simulink model "FPU_sim1"  (Simulink 7.6)
settings: Solver=FixedStepDiscrete  StartTime=0.0  StopTime=6000  FixedStep=1  RelTol=1e-3
values from neighbouring files (symbols this model uses):
  data_init_sim = zeros(1,100)    [Init_mem.m]    (also in exp_doc.mat = [0 0 0 0 0 0 986822423 3304964096 1146115413 1152155648 1065)
  out_file = [out_file; ['5' buf_oper]]    [Convert_IVE_Program.m]    (also in exp_doc.mat = '78383136191212713131367131313671313136197131361950000000000)
libraries: simulink x50
settings Model: Creator=jordan  LastModifiedBy=jordan
settings OptimizationCC: BlockReduction=off  ConditionallyExecuteInputs=off

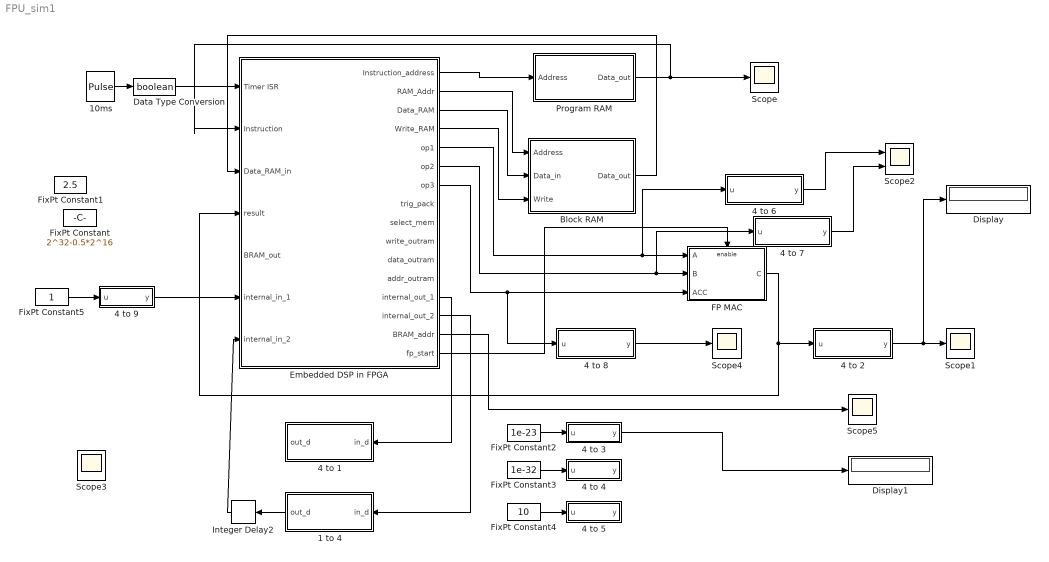
== system FPU_sim1 ==
  1 to 4 : Stateflow chart  TreatAsAtomicUnit=on
  10ms : DiscretePulseGenerator  Period=3000
  4 to 1 : Stateflow chart  TreatAsAtomicUnit=on
  4 to 2 : Stateflow chart  TreatAsAtomicUnit=on
  4 to 3 : Stateflow chart  TreatAsAtomicUnit=on
  4 to 4 : Stateflow chart  TreatAsAtomicUnit=on
  4 to 5 : Stateflow chart  TreatAsAtomicUnit=on
  4 to 6 : Stateflow chart  TreatAsAtomicUnit=on
  4 to 7 : Stateflow chart  TreatAsAtomicUnit=on
  4 to 8 : Stateflow chart  TreatAsAtomicUnit=on
  4 to 9 : Stateflow chart  TreatAsAtomicUnit=on
  Block RAM : Subsystem
  Data Type Conversion : DataTypeConversion  OutDataTypeStr=boolean
  Display : Display
  Display1 : Display
  Embedded DSP in FPGA : Subsystem
  FP MAC : Subsystem
  FixPt Constant : Constant  DisableCoverage=on  Value=2^32-0.5*2^16  OutDataTypeStr=uint32
  FixPt Constant1 : Constant  DisableCoverage=on  Value=2.5  OutDataTypeStr=fixdt(1,32,16)  LockScale=on
  FixPt Constant2 : Constant  DisableCoverage=on  Value=1e-23  OutDataTypeStr=single  LockScale=on
  FixPt Constant3 : Constant  DisableCoverage=on  Value=1e-32  OutDataTypeStr=single  LockScale=on
  FixPt Constant4 : Constant  DisableCoverage=on  Value=10  OutDataTypeStr=single  LockScale=on
  FixPt Constant5 : Constant  DisableCoverage=on  OutDataTypeStr=single  LockScale=on
  Integer Delay2 : simulink/Discrete/Integer Delay  NumDelays=1  vinit=0.0  samptime=-1
  Program RAM : Subsystem
  Scope{,1,3..5} (5 alike) : Scope
      Scope settings: MaxDataPoints=50000
      Scope1 settings: SaveName=ScopeData3  MaxDataPoints=50000
      Scope3 settings: SaveName=ScopeData19  MaxDataPoints=50000
      Scope4 settings: SaveName=ScopeData5  MaxDataPoints=50000
      Scope5 settings: SaveName=ScopeData11  MaxDataPoints=50000
  Scope2 : Scope  NumInputPorts=2
      settings: YMin=-5~-5  YMax=5~5  SaveName=ScopeData4  MaxDataPoints=50000
  wires:
  10ms/1 -> Data Type Conversion/1
  Program RAM/1(Data_out) -> Scope/1, Embedded DSP in FPGA/2(Instruction)
  1 to 4/1(out_d) -> Integer Delay2/1
  Data Type Conversion/1 -> Embedded DSP in FPGA/1(Timer ISR)
  Block RAM/1(Data_out) -> Embedded DSP in FPGA/3(Data_RAM_in)
  Embedded DSP in FPGA/13(internal_out_1) -> 4 to 1/1(in_d)
  Embedded DSP in FPGA/14(internal_out_2) -> 1 to 4/1(in_d)
  Integer Delay2/1 -> Embedded DSP in FPGA/7(internal_in_2)
  Embedded DSP in FPGA/1(Instruction_address) -> Program RAM/1(Address)
  Embedded DSP in FPGA/2(RAM_Addr) -> Block RAM/1(Address)
  Embedded DSP in FPGA/3(Data_RAM) -> Block RAM/2(Data_in)
  Embedded DSP in FPGA/4(Write_RAM) -> Block RAM/3(Write)
  Embedded DSP in FPGA/5(op1) -> 4 to 6/1(u), FP MAC/1(A)
  Embedded DSP in FPGA/6(op2) -> FP MAC/2(B), 4 to 7/1(u)
  Embedded DSP in FPGA/7(op3) -> FP MAC/3(ACC), 4 to 8/1(u)
  FP MAC/1(C) -> Embedded DSP in FPGA/4(result), 4 to 2/1(u)
  4 to 2/1(y) -> Scope1/1, Display/1
  FixPt Constant2/1 -> 4 to 3/1(u)
  4 to 3/1(y) -> Display1/1
  FixPt Constant3/1 -> 4 to 4/1(u)
  FixPt Constant4/1 -> 4 to 5/1(u)
  4 to 6/1(y) -> Scope2/1
  4 to 7/1(y) -> Scope2/2
  4 to 8/1(y) -> Scope4/1
  4 to 9/1(y) -> Embedded DSP in FPGA/6(internal_in_1)
  FixPt Constant5/1 -> 4 to 9/1(u)
  Embedded DSP in FPGA/16(fp_start) -> FP MAC/Enable
  Embedded DSP in FPGA/15(BRAM_addr) -> Scope5/1

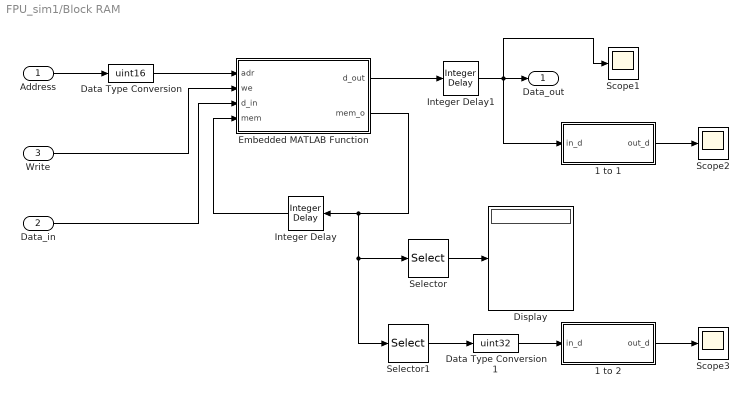
== system FPU_sim1/Block RAM ==
  Address : Inport  OutDataTypeStr=fixdt(0,12,0)
  Data_in : Inport  Port=2  OutDataTypeStr=uint32
  Write : Inport  Port=3  OutDataTypeStr=boolean
  1 to 1 : Stateflow chart  TreatAsAtomicUnit=on
  1 to 2 : Stateflow chart  TreatAsAtomicUnit=on
  Data Type Conversion : DataTypeConversion  OutDataTypeStr=uint16
  Data Type Conversion1 : DataTypeConversion  OutDataTypeStr=uint32
  Display : Display
  Embedded MATLAB Function : Stateflow chart  TreatAsAtomicUnit=on
  Integer Delay : simulink/Discrete/Integer Delay  NumDelays=1  vinit=data_init_sim  samptime=-1
  Integer Delay1 : simulink/Discrete/Integer Delay  NumDelays=1  vinit=0.0  samptime=-1
  Scope1 : Scope
      settings: SaveName=ScopeData23  MaxDataPoints=50000
  Scope2 : Scope
      settings: SaveName=ScopeData14  MaxDataPoints=50000
  Scope3 : Scope
      settings: SaveName=ScopeData31  MaxDataPoints=50000
  Selector : Selector  InputPortWidth=2048  IndexOptions=Index vector (dialog)  Indices=1:5  OutputSizes=1
  Selector1 : Selector  InputPortWidth=2048  IndexOptions=Index vector (dialog)  Indices=37  OutputSizes=1
  Data_out : Outport  OutDataTypeStr=uint32
  wires:
  Address/1 -> Data Type Conversion/1
  Write/1 -> Embedded MATLAB Function/2(we)
  Data_in/1 -> Embedded MATLAB Function/3(d_in)
  Embedded MATLAB Function/1(d_out) -> Integer Delay1/1
  Integer Delay/1 -> Embedded MATLAB Function/4(mem)
  Embedded MATLAB Function/2(mem_o) -> Integer Delay/1, Selector/1, Selector1/1
  Data Type Conversion/1 -> Embedded MATLAB Function/1(adr)
  Integer Delay1/1 -> Data_out/1, Scope1/1, 1 to 1/1(in_d)
  Selector/1 -> Display/1
  1 to 1/1(out_d) -> Scope2/1
  1 to 2/1(out_d) -> Scope3/1
  Selector1/1 -> Data Type Conversion1/1
  Data Type Conversion1/1 -> 1 to 2/1(in_d)

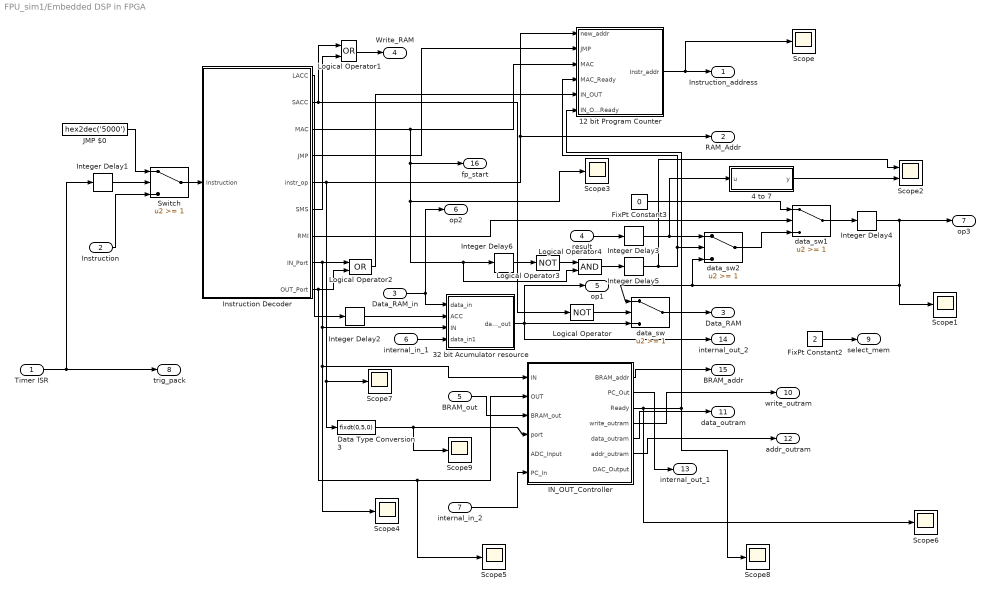
== system FPU_sim1/Embedded DSP in FPGA ==
  Timer ISR : Inport  OutDataTypeStr=boolean
  Instruction : Inport  Port=2  OutDataTypeStr=uint16
  Data_RAM_in : Inport  Port=3  OutDataTypeStr=uint32
  result : Inport  Port=4  OutDataTypeStr=uint32
  BRAM_out : Inport  Port=5  OutDataTypeStr=uint8
  internal_in_1 : Inport  Port=6  OutDataTypeStr=uint32
  internal_in_2 : Inport  Port=7  OutDataTypeStr=uint8  PortDimensions=4
  12 bit Program Counter : Subsystem
  32 bit Acumulator resource : Subsystem
  4 to 7 : Stateflow chart  TreatAsAtomicUnit=on
  Data Type Conversion3 : DataTypeConversion  OutDataTypeStr=fixdt(0,5,0)
  FixPt Constant2 : Constant  DisableCoverage=on  Value=2  OutDataTypeStr=fixdt(0,4,0)
  FixPt Constant3 : Constant  DisableCoverage=on  Value=0  OutDataTypeStr=uint32
  IN_OUT_Controller : Subsystem
  Instruction Decoder : Subsystem
  Integer Delay{1..4,6} (5 alike) : simulink/Discrete/Integer Delay  NumDelays=1  vinit=0.0  samptime=-1
  Integer Delay5 : simulink/Discrete/Integer Delay  NumDelays=3  vinit=0.0  samptime=-1
  JMP $0 : Constant  DisableCoverage=on  Value=hex2dec('5000')  OutDataTypeStr=Inherit: Inherit via back propagation
  Logical Operator : Logic  Operator=NOT  AllPortsSameDT=off  OutDataTypeStr=boolean
  Logical Operator1 : Logic  Operator=OR  AllPortsSameDT=off  OutDataTypeStr=boolean
  Logical Operator2 : Logic  Operator=OR  AllPortsSameDT=off  OutDataTypeStr=boolean
  Logical Operator3 : Logic  Operator=NOT  AllPortsSameDT=off  OutDataTypeStr=boolean
  Logical Operator4 : Logic  AllPortsSameDT=off  OutDataTypeStr=boolean
  Scope{,1,3..9} (9 alike) : Scope
      Scope settings: YMin=0  YMax=650  SaveName=ScopeData2  MaxDataPoints=50000
      Scope1 settings: SaveName=ScopeData6  MaxDataPoints=50000
      Scope3 settings: SaveName=ScopeData8  MaxDataPoints=50000
      Scope4 settings: SaveName=ScopeData10  MaxDataPoints=50000
      Scope5 settings: SaveName=ScopeData21  MaxDataPoints=50000
      Scope6 settings: SaveName=ScopeData13  MaxDataPoints=50000
      Scope7 settings: SaveName=ScopeData15  MaxDataPoints=50000
      Scope8 settings: SaveName=ScopeData16  MaxDataPoints=50000
      Scope9 settings: SaveName=ScopeData12  MaxDataPoints=50000
  Scope2 : Scope  NumInputPorts=2
      settings: YMin=-5~-5  YMax=5~5  SaveName=ScopeData7  MaxDataPoints=50000
  Switch : Switch  Threshold=1
  data_sw : Switch  Threshold=1
  data_sw1 : Switch  Threshold=1
  data_sw2 : Switch  Threshold=1
  Instruction_address : Outport  OutDataTypeStr=fixdt(0,12,0)
  RAM_Addr : Outport  Port=2  OutDataTypeStr=fixdt(0,12,0)
  Data_RAM : Outport  Port=3  OutDataTypeStr=uint32
  Write_RAM : Outport  Port=4  OutDataTypeStr=boolean
  op1 : Outport  Port=5  OutDataTypeStr=uint32
  op2 : Outport  Port=6  OutDataTypeStr=uint32
  op3 : Outport  Port=7  OutDataTypeStr=uint32
  trig_pack : Outport  Port=8
  select_mem : Outport  Port=9
  write_outram : Outport  Port=10
  data_outram : Outport  Port=11
  addr_outram : Outport  Port=12
  internal_out_1 : Outport  Port=13
  internal_out_2 : Outport  Port=14  OutDataTypeStr=uint32
  BRAM_addr : Outport  Port=15
  fp_start : Outport  Port=16  OutDataTypeStr=boolean
  wires:
  32 bit Acumulator resource/1(data_out) -> data_sw/3, op1/1, internal_out_2/1
  Data_RAM_in/1 -> 32 bit Acumulator resource/1(data_in), op2/1
  Instruction Decoder/5(instr_op) -> 12 bit Program Counter/1(new_addr), RAM_Addr/1, Data Type Conversion3/1, Scope7/1
  Instruction Decoder/1(LACC) -> Integer Delay2/1
  Integer Delay2/1 -> 32 bit Acumulator resource/2(ACC)
  Instruction Decoder/2(SACC) -> Logical Operator/1, Logical Operator1/1
  Logical Operator/1 -> data_sw/2
  Instruction Decoder/4(JMP) -> 12 bit Program Counter/2(JMP)
  Instruction Decoder/3(MAC) -> 12 bit Program Counter/3(MAC), fp_start/1, Logical Operator4/2, Integer Delay6/1, Scope3/1
  Instruction Decoder/7(RMI) -> data_sw1/2
  Instruction Decoder/6(SMS) -> Logical Operator1/2
  Instruction Decoder/8(IN_Port) -> 32 bit Acumulator resource/3(IN), Scope4/1, IN_OUT_Controller/1(IN), Logical Operator2/1
  Data Type Conversion3/1 -> Scope9/1, IN_OUT_Controller/4(port)
  Switch/1 -> Instruction Decoder/1(Instruction)
  JMP $0/1 -> Switch/1
  12 bit Program Counter/1(Instr_addr) -> Instruction_address/1, Scope/1
  Instruction/1 -> Switch/3
  data_sw/1 -> Data_RAM/1
  Logical Operator1/1 -> Write_RAM/1
  result/1 -> Integer Delay3/1
  Instruction Decoder/9(OUT_Port) -> Logical Operator2/2, Scope5/1, IN_OUT_Controller/2(OUT)
  IN_OUT_Controller/4(write_outram) -> write_outram/1
  IN_OUT_Controller/5(data_outram) -> data_outram/1
  IN_OUT_Controller/3(Ready) -> 12 bit Program Counter/6(IN_OUT_Ready), Scope8/1, Scope6/1
  Logical Operator2/1 -> 12 bit Program Counter/5(IN_OUT)
  internal_in_1/1 -> 32 bit Acumulator resource/4(data_in1)
  internal_in_2/1 -> IN_OUT_Controller/6(PC_In)
  Integer Delay1/1 -> Switch/2
  IN_OUT_Controller/2(PC_Out) -> internal_out_1/1
  IN_OUT_Controller/1(BRAM_addr) -> BRAM_addr/1
  FixPt Constant2/1 -> select_mem/1
  Timer ISR/1 -> trig_pack/1, Integer Delay1/1
  Integer Delay4/1 -> data_sw2/3, data_sw/1, Scope1/1, op3/1
  data_sw1/1 -> Integer Delay4/1
  FixPt Constant3/1 -> data_sw1/1
  data_sw2/1 -> data_sw1/3
  Integer Delay3/1 -> data_sw2/1, 4 to 7/1(u)
  4 to 7/1(y) -> Scope2/2
  Integer Delay5/1 -> 12 bit Program Counter/4(MAC_Ready), data_sw2/2, Scope2/1
  Integer Delay6/1 -> Logical Operator3/1
  Logical Operator3/1 -> Logical Operator4/1
  Logical Operator4/1 -> Integer Delay5/1
  IN_OUT_Controller/6(addr_outram) -> addr_outram/1
  BRAM_out/1 -> IN_OUT_Controller/3(BRAM_out)

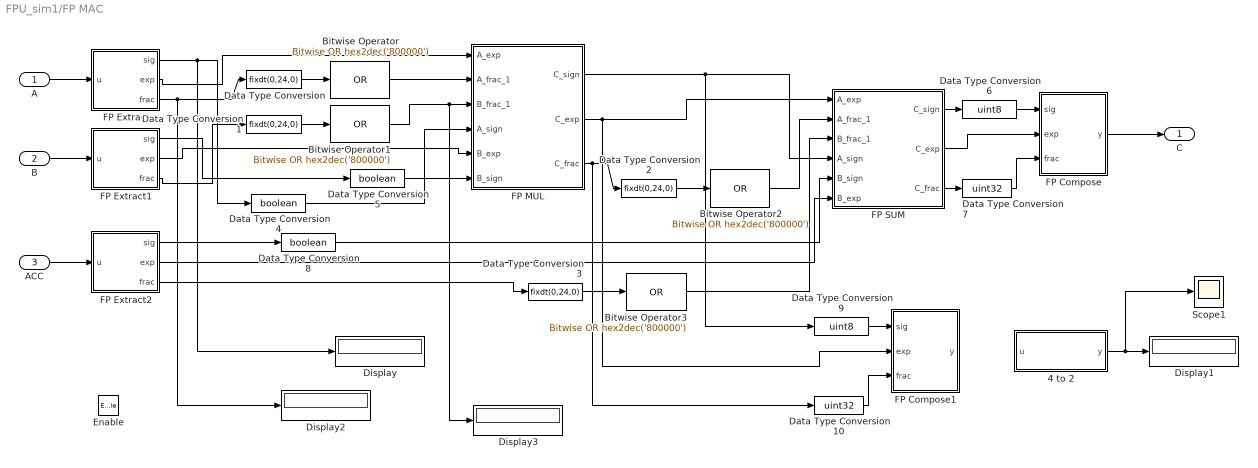
== system FPU_sim1/FP MAC ==
  A : Inport
  B : Inport  Port=2
  ACC : Inport  Port=3
  Enable : EnablePort
  4 to 2 : Stateflow chart  TreatAsAtomicUnit=on
  Bitwise Operator{,1..3} (4 alike) : simulink/Logic and Bit Operations/Bitwise Operator  logicop=OR  UseBitMask=on  BitMask=hex2dec('800000')  BitMaskRealWorld=Stored Integer
  Data Type Conversion{,1..3} (4 alike) : DataTypeConversion  OutDataTypeStr=fixdt(0,24,0)  RndMeth=Nearest
  Data Type Conversion10 : DataTypeConversion  OutDataTypeStr=uint32  RndMeth=Nearest
  Data Type Conversion4 : DataTypeConversion  OutDataTypeStr=boolean  RndMeth=Nearest
  Data Type Conversion5 : DataTypeConversion  OutDataTypeStr=boolean  RndMeth=Nearest
  Data Type Conversion6 : DataTypeConversion  OutDataTypeStr=uint8  RndMeth=Nearest
  Data Type Conversion7 : DataTypeConversion  OutDataTypeStr=uint32  RndMeth=Nearest
  Data Type Conversion8 : DataTypeConversion  OutDataTypeStr=boolean  RndMeth=Nearest
  Data Type Conversion9 : DataTypeConversion  OutDataTypeStr=uint8  RndMeth=Nearest
  Display{,1..3} (4 alike) : Display
      Display3 settings: Format=hex (Stored Integer)
  FP Compose : Stateflow chart  TreatAsAtomicUnit=on
  FP Compose1 : Stateflow chart  TreatAsAtomicUnit=on
  FP Extract : Stateflow chart  TreatAsAtomicUnit=on
  FP Extract1 : Stateflow chart  TreatAsAtomicUnit=on
  FP Extract2 : Stateflow chart  TreatAsAtomicUnit=on
  FP MUL : Subsystem
  FP SUM : Subsystem
  Scope1 : Scope
      settings: SaveName=ScopeData9  MaxDataPoints=50000
  C : Outport  InitialOutput=0
  wires:
  A/1 -> FP Extract/1(u)
  B/1 -> FP Extract1/1(u)
  ACC/1 -> FP Extract2/1(u)
  FP Extract/1(sig) -> Data Type Conversion4/1, Display/1
  FP Extract1/1(sig) -> Data Type Conversion5/1
  FP Extract/2(exp) -> FP MUL/1(A_exp)
  FP Extract1/2(exp) -> FP MUL/5(B_exp)
  FP Extract/3(frac) -> Data Type Conversion/1, Display2/1
  FP Extract1/3(frac) -> Data Type Conversion1/1
  Data Type Conversion/1 -> Bitwise Operator/1
  Bitwise Operator/1 -> FP MUL/2(A_frac_1)
  Data Type Conversion1/1 -> Bitwise Operator1/1
  Bitwise Operator1/1 -> FP MUL/3(B_frac_1), Display3/1
  FP MUL/1(C_sign) -> FP SUM/4(A_sign), Data Type Conversion9/1
  FP MUL/2(C_exp) -> FP SUM/1(A_exp), FP Compose1/2(exp)
  FP MUL/3(C_frac) -> Data Type Conversion2/1, Data Type Conversion10/1
  Data Type Conversion2/1 -> Bitwise Operator2/1
  Bitwise Operator2/1 -> FP SUM/2(A_frac_1)
  FP Extract2/1(sig) -> Data Type Conversion8/1
  FP Extract2/2(exp) -> FP SUM/6(B_exp)
  FP Extract2/3(frac) -> Data Type Conversion3/1
  Data Type Conversion3/1 -> Bitwise Operator3/1
  Bitwise Operator3/1 -> FP SUM/3(B_frac_1)
  Data Type Conversion4/1 -> FP MUL/4(A_sign)
  Data Type Conversion5/1 -> FP MUL/6(B_sign)
  FP SUM/1(C_sign) -> Data Type Conversion6/1
  FP SUM/2(C_exp) -> FP Compose/2(exp)
  FP SUM/3(C_frac) -> Data Type Conversion7/1
  FP Compose/1(y) -> C/1
  Data Type Conversion6/1 -> FP Compose/1(sig)
  Data Type Conversion7/1 -> FP Compose/3(frac)
  Data Type Conversion8/1 -> FP SUM/5(B_sign)
  Data Type Conversion9/1 -> FP Compose1/1(sig)
  Data Type Conversion10/1 -> FP Compose1/3(frac)
  4 to 2/1(y) -> Display1/1, Scope1/1

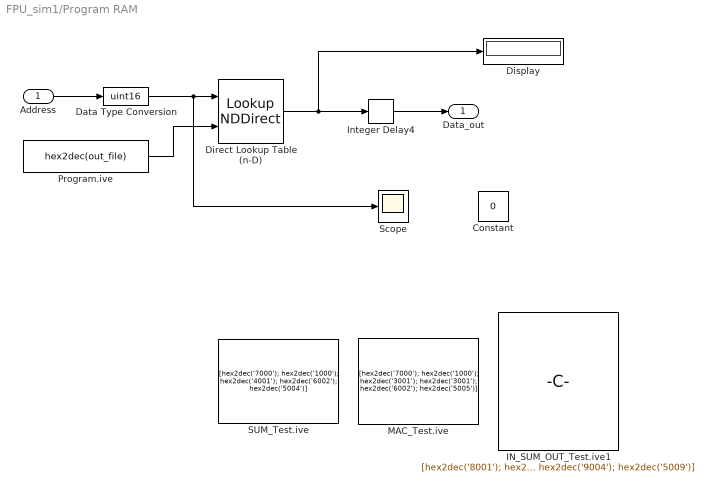
== system FPU_sim1/Program RAM ==
  Address : Inport
  Constant : Constant  Value=0
  Data Type Conversion : DataTypeConversion  OutDataTypeStr=uint16
  Direct Lookup Table (n-D) : LookupNDDirect  NumberOfTableDimensions=1  TableIsInput=on  Table=[hex2dec('1000') hex2dec('4001') hex2dec('2002') hex2dec('5003')]  SampleTime=1  TableDataTypeStr=uint16
  Display : Display
      settings: Format=hex (Stored Integer)
  IN_SUM_OUT_Test.ive1 : Constant  Value=[hex2dec('8001'); hex2dec('2000'); hex2dec('8002'); hex2dec('2001'); hex2dec('1000'); hex2dec('4001'); hex2dec('6002'); hex2dec('1002'); hex2dec('9004'); hex2dec('5009')]  VectorParams1D=off  OutDataTypeStr=uint16
  Integer Delay4 : simulink/Discrete/Integer Delay  NumDelays=1  vinit=0.0  samptime=-1
  MAC_Test.ive : Constant  Value=[hex2dec('7000'); hex2dec('1000'); hex2dec('3001'); hex2dec('3001'); hex2dec('6002'); hex2dec('5005')]  VectorParams1D=off  OutDataTypeStr=uint16
  Program.ive : Constant  Value=hex2dec(out_file)  VectorParams1D=off  OutDataTypeStr=uint16
  SUM_Test.ive : Constant  Value=[hex2dec('7000'); hex2dec('1000'); hex2dec('4001'); hex2dec('6002'); hex2dec('5004')]  VectorParams1D=off  OutDataTypeStr=uint16
  Scope : Scope
      settings: MaxDataPoints=50000
  Data_out : Outport
  wires:
  Address/1 -> Data Type Conversion/1
  Direct Lookup Table (n-D)/1 -> Display/1, Integer Delay4/1
  Program.ive/1 -> Direct Lookup Table (n-D)/2
  Integer Delay4/1 -> Data_out/1
  Data Type Conversion/1 -> Direct Lookup Table (n-D)/1, Scope/1

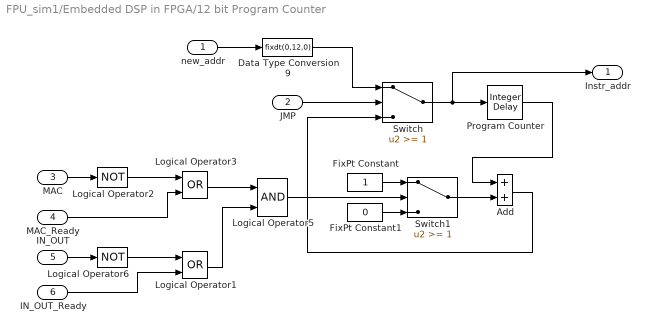
== system FPU_sim1/Embedded DSP in FPGA/12 bit Program Counter ==
  new_addr : Inport
  JMP : Inport  Port=2
  MAC : Inport  Port=3  OutDataTypeStr=boolean
  MAC_Ready : Inport  Port=4  OutDataTypeStr=boolean
  IN_OUT : Inport  Port=5  OutDataTypeStr=boolean
  IN_OUT_Ready : Inport  Port=6  OutDataTypeStr=boolean
  Add : Sum  AccumDataTypeStr=fixdt(0,12,0)  OutDataTypeStr=fixdt(0,12,0)
  Data Type Conversion9 : DataTypeConversion  OutDataTypeStr=fixdt(0,12,0)
  FixPt Constant : Constant  DisableCoverage=on  OutDataTypeStr=fixdt(0,12,0)
  FixPt Constant1 : Constant  DisableCoverage=on  Value=0  OutDataTypeStr=fixdt(0,12,0)
  Logical Operator1 : Logic  Operator=OR  AllPortsSameDT=off  OutDataTypeStr=boolean
  Logical Operator2 : Logic  Operator=NOT  AllPortsSameDT=off  OutDataTypeStr=boolean
  Logical Operator3 : Logic  Operator=OR  AllPortsSameDT=off  OutDataTypeStr=boolean
  Logical Operator5 : Logic  AllPortsSameDT=off  OutDataTypeStr=boolean
  Logical Operator6 : Logic  Operator=NOT  AllPortsSameDT=off  OutDataTypeStr=boolean
  Program Counter : simulink/Discrete/Integer Delay  NumDelays=1  vinit=0.0  samptime=-1
  Switch : Switch  Threshold=1
  Switch1 : Switch  Threshold=1
  Instr_addr : Outport  InitialOutput=0
  wires:
  JMP/1 -> Switch/2
  new_addr/1 -> Data Type Conversion9/1
  Program Counter/1 -> Add/1
  Switch/1 -> Program Counter/1, Instr_addr/1
  FixPt Constant/1 -> Switch1/1
  Add/1 -> Switch/3
  Data Type Conversion9/1 -> Switch/1
  Switch1/1 -> Add/2
  FixPt Constant1/1 -> Switch1/3
  Logical Operator3/1 -> Logical Operator5/1
  Logical Operator2/1 -> Logical Operator3/1
  MAC/1 -> Logical Operator2/1
  Logical Operator1/1 -> Logical Operator5/2
  Logical Operator6/1 -> Logical Operator1/1
  IN_OUT/1 -> Logical Operator6/1
  IN_OUT_Ready/1 -> Logical Operator1/2
  Logical Operator5/1 -> Switch1/2
  MAC_Ready/1 -> Logical Operator3/2

== system FPU_sim1/Embedded DSP in FPGA/32 bit Acumulator resource ==
  data_in : Inport
  ACC : Inport  Port=2
  IN : Inport  Port=3
  data_in1 : Inport  Port=4
  Integer Delay2 : simulink/Discrete/Integer Delay  NumDelays=1  vinit=0.0  samptime=-1
  Switch : Switch  Threshold=1
  Switch1 : Switch  Threshold=1
  data_out : Outport  OutDataTypeStr=uint32
  wires:
  Switch/1 -> Switch1/3
  Integer Delay2/1 -> Switch/3
  data_in/1 -> Switch/1
  ACC/1 -> Switch/2
  Switch1/1 -> Integer Delay2/1, data_out/1
  IN/1 -> Switch1/2
  data_in1/1 -> Switch1/1

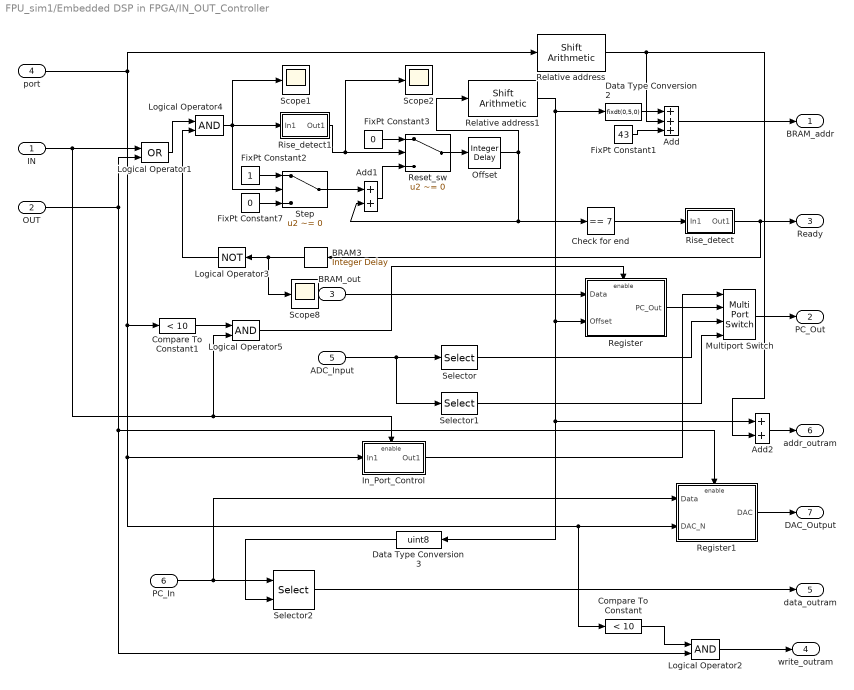
== system FPU_sim1/Embedded DSP in FPGA/IN_OUT_Controller ==
  IN : Inport  OutDataTypeStr=boolean
  OUT : Inport  Port=2  OutDataTypeStr=boolean
  BRAM_out : Inport  Port=3  OutDataTypeStr=uint8
  port : Inport  Port=4  OutDataTypeStr=fixdt(0,5,0)
  ADC_Input : Inport  Port=5  OutDataTypeStr=uint8  PortDimensions=8
  PC_In : Inport  Port=6  OutDataTypeStr=uint8  PortDimensions=4
  Add : Sum  Inputs=+++  AccumDataTypeStr=fixdt(0,11,0)  OutDataTypeStr=fixdt(0,11,0)  SaturateOnIntegerOverflow=on
  Add1 : Sum  AccumDataTypeStr=fixdt(0,3,0)  OutDataTypeStr=fixdt(0,3,0)  SaturateOnIntegerOverflow=on
  Add2 : Sum  AccumDataTypeStr=fixdt(0,14,0)  OutDataTypeStr=fixdt(0,14,0)
  BRAM3 : simulink/Discrete/Integer Delay  NumDelays=1  vinit=0.0  samptime=-1
  Check for end : simulink/Logic and Bit Operations/Compare To Constant  SystemSampleTime=-1  relop===  const=7  LogicOutDataTypeMode=boolean
  Compare To Constant : simulink/Logic and Bit Operations/Compare To Constant  SystemSampleTime=-1  relop=<  const=10  LogicOutDataTypeMode=boolean
  Compare To Constant1 : simulink/Logic and Bit Operations/Compare To Constant  SystemSampleTime=-1  relop=<  const=10  LogicOutDataTypeMode=boolean
  Data Type Conversion2 : DataTypeConversion  OutDataTypeStr=fixdt(0,5,0)
  Data Type Conversion3 : DataTypeConversion  OutDataTypeStr=uint8
  FixPt Constant1 : Constant  DisableCoverage=on  Value=43  OutDataTypeStr=fixdt(0,11,0)
  FixPt Constant2 : Constant  DisableCoverage=on  OutDataTypeStr=fixdt(0,3,0)
  FixPt Constant3 : Constant  DisableCoverage=on  Value=0  OutDataTypeStr=fixdt(0,3,0)
  FixPt Constant7 : Constant  DisableCoverage=on  Value=0  OutDataTypeStr=fixdt(0,3,0)
  In_Port_Control : Subsystem
  Logical Operator1 : Logic  Operator=OR  AllPortsSameDT=off  OutDataTypeStr=boolean
  Logical Operator2 : Logic  AllPortsSameDT=off  OutDataTypeStr=boolean
  Logical Operator3 : Logic  Operator=NOT  AllPortsSameDT=off  OutDataTypeStr=boolean
  Logical Operator4 : Logic  AllPortsSameDT=off  OutDataTypeStr=boolean
  Logical Operator5 : Logic  AllPortsSameDT=off  OutDataTypeStr=boolean
  Multiport Switch : MultiPortSwitch  DataPortOrder=Zero-based contiguous  zeroidx=on
  Offset : simulink/Discrete/Integer Delay  NumDelays=1  vinit=0.0  samptime=0
  Register : Subsystem
  Register1 : Subsystem
  Relative address : simulink/Logic and Bit Operations/Shift Arithmetic  SystemSampleTime=-1  nBitShiftRight=-2  nBinPtShiftRight=0
  Relative address1 : simulink/Logic and Bit Operations/Shift Arithmetic  SystemSampleTime=-1  nBitShiftRight=1  nBinPtShiftRight=0
  Reset_sw : Switch  Criteria=u2 ~= 0
  Rise_detect : Subsystem
  Rise_detect1 : Subsystem
  Scope1 : Scope
      settings: SaveName=ScopeData18  MaxDataPoints=50000
  Scope2 : Scope
      settings: SaveName=ScopeData20  MaxDataPoints=50000
  Scope8 : Scope
      settings: SaveName=ScopeData17  MaxDataPoints=50000
  Selector : Selector  InputPortWidth=8  IndexOptions=Index vector (dialog)  Indices=1:4  OutputSizes=1
  Selector1 : Selector  InputPortWidth=8  IndexOptions=Index vector (dialog)  Indices=5:8  OutputSizes=1
  Selector2 : Selector  IndexMode=Zero-based  InputPortWidth=4  IndexOptions=Index vector (port)  Indices=5:8  OutputSizes=1
  Step : Switch  Criteria=u2 ~= 0
  BRAM_addr : Outport
  PC_Out : Outport  Port=2  OutDataTypeStr=uint8  PortDimensions=4
  Ready : Outport  Port=3
  write_outram : Outport  Port=4
  data_outram : Outport  Port=5
  addr_outram : Outport  Port=6
  DAC_Output : Outport  Port=7  OutDataTypeStr=uint8  PortDimensions=8
  wires:
  Register1/1(DAC) -> DAC_Output/1
  OUT/1 -> Logical Operator1/2, Logical Operator2/2, Register1/Enable
  IN/1 -> Logical Operator1/1, In_Port_Control/Enable, Logical Operator5/2
  Selector2/1 -> data_outram/1
  PC_In/1 -> Selector2/1, Register1/1(Data)
  Add2/1 -> addr_outram/1
  BRAM_out/1 -> Register/1(Data)
  FixPt Constant7/1 -> Step/3
  Step/1 -> Add1/1
  In_Port_Control/1(Out1) -> Multiport Switch/1
  Selector1/1 -> Multiport Switch/4
  ADC_Input/1 -> Selector1/1, Selector/1
  Selector/1 -> Multiport Switch/3
  Multiport Switch/1 -> PC_Out/1
  Check for end/1 -> Rise_detect/1(In1)
  FixPt Constant3/1 -> Reset_sw/1
  Rise_detect1/1(Out1) -> Reset_sw/2, Scope2/1
  Register/1(PC_Out) -> Multiport Switch/2
  Logical Operator4/1 -> Rise_detect1/1(In1), Step/2, Scope1/1
  port/1 -> Relative address/1, In_Port_Control/1(In1), Register1/2(DAC_N), Compare To Constant/1, Compare To Constant1/1
  Relative address/1 -> Add2/2, Add/2
  FixPt Constant2/1 -> Step/1
  Add1/1 -> Reset_sw/3
  Reset_sw/1 -> Offset/1
  FixPt Constant1/1 -> Add/3
  Data Type Conversion2/1 -> Add/1
  Add/1 -> BRAM_addr/1
  Offset/1 -> Relative address1/1, Add1/2, Check for end/1
  Rise_detect/1(Out1) -> Ready/1, BRAM3/1
  Data Type Conversion3/1 -> Selector2/2
  Relative address1/1 -> Data Type Conversion2/1, Register/2(Offset), Add2/1, Data Type Conversion3/1
  Logical Operator2/1 -> write_outram/1
  Compare To Constant/1 -> Logical Operator2/1
  Logical Operator3/1 -> Logical Operator4/2
  Logical Operator1/1 -> Logical Operator4/1
  Logical Operator5/1 -> Register/Enable
  Compare To Constant1/1 -> Logical Operator5/1
  BRAM3/1 -> Logical Operator3/1, Scope8/1

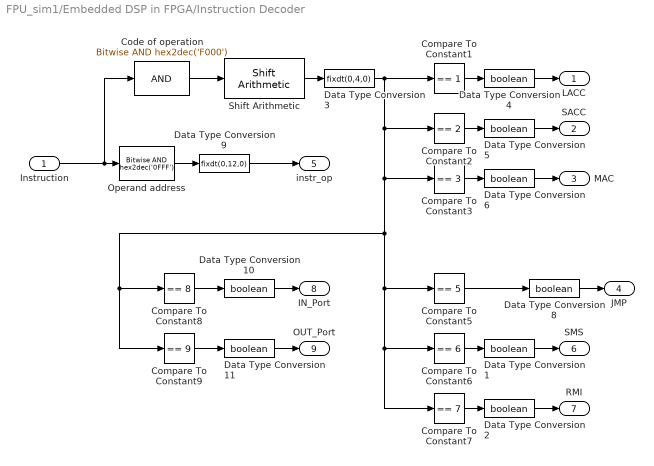
== system FPU_sim1/Embedded DSP in FPGA/Instruction Decoder ==
  Instruction : Inport  OutDataTypeStr=uint16
  Code of operation : simulink/Logic and Bit Operations/Bitwise Operator  logicop=AND  UseBitMask=on  BitMask=hex2dec('F000')  BitMaskRealWorld=Stored Integer
  Compare To Constant1 : simulink/Logic and Bit Operations/Compare To Constant  SystemSampleTime=-1  relop===  const=1  LogicOutDataTypeMode=boolean
  Compare To Constant2 : simulink/Logic and Bit Operations/Compare To Constant  SystemSampleTime=-1  relop===  const=2  LogicOutDataTypeMode=boolean
  Compare To Constant3 : simulink/Logic and Bit Operations/Compare To Constant  SystemSampleTime=-1  relop===  const=3  LogicOutDataTypeMode=boolean
  Compare To Constant5 : simulink/Logic and Bit Operations/Compare To Constant  SystemSampleTime=-1  relop===  const=5  LogicOutDataTypeMode=boolean
  Compare To Constant6 : simulink/Logic and Bit Operations/Compare To Constant  SystemSampleTime=-1  relop===  const=6  LogicOutDataTypeMode=boolean
  Compare To Constant7 : simulink/Logic and Bit Operations/Compare To Constant  SystemSampleTime=-1  relop===  const=7  LogicOutDataTypeMode=boolean
  Compare To Constant8 : simulink/Logic and Bit Operations/Compare To Constant  SystemSampleTime=-1  relop===  const=8  LogicOutDataTypeMode=boolean
  Compare To Constant9 : simulink/Logic and Bit Operations/Compare To Constant  SystemSampleTime=-1  relop===  const=9  LogicOutDataTypeMode=boolean
  Data Type Conversion{1..2,4..6,8,10..11} (8 alike) : DataTypeConversion  OutDataTypeStr=boolean
  Data Type Conversion3 : DataTypeConversion  OutDataTypeStr=fixdt(0,4,0)
  Data Type Conversion9 : DataTypeConversion  OutDataTypeStr=fixdt(0,12,0)
  Operand address : simulink/Logic and Bit Operations/Bitwise Operator  logicop=AND  UseBitMask=on  BitMask=hex2dec('0FFF')  BitMaskRealWorld=Stored Integer
  Shift Arithmetic : simulink/Logic and Bit Operations/Shift Arithmetic  SystemSampleTime=-1  nBitShiftRight=12  nBinPtShiftRight=0
  LACC : Outport
  SACC : Outport  Port=2
  MAC : Outport  Port=3
  JMP : Outport  Port=4
  instr_op : Outport  Port=5
  SMS : Outport  Port=6
  RMI : Outport  Port=7
  IN_Port : Outport  Port=8
  OUT_Port : Outport  Port=9
  wires:
  Instruction/1 -> Operand address/1, Code of operation/1
  Code of operation/1 -> Shift Arithmetic/1
  Shift Arithmetic/1 -> Data Type Conversion3/1
  Data Type Conversion3/1 -> Compare To Constant6/1, Compare To Constant7/1, Compare To Constant5/1, Compare To Constant8/1, Compare To Constant9/1, Compare To Constant3/1, Compare To Constant2/1, Compare To Constant1/1
  Compare To Constant1/1 -> Data Type Conversion4/1
  Compare To Constant2/1 -> Data Type Conversion5/1
  Compare To Constant3/1 -> Data Type Conversion6/1
  Compare To Constant5/1 -> Data Type Conversion8/1
  Operand address/1 -> Data Type Conversion9/1
  Data Type Conversion4/1 -> LACC/1
  Data Type Conversion5/1 -> SACC/1
  Data Type Conversion9/1 -> instr_op/1
  Data Type Conversion6/1 -> MAC/1
  Data Type Conversion8/1 -> JMP/1
  Compare To Constant6/1 -> Data Type Conversion1/1
  Data Type Conversion1/1 -> SMS/1
  Compare To Constant7/1 -> Data Type Conversion2/1
  Data Type Conversion2/1 -> RMI/1
  Compare To Constant8/1 -> Data Type Conversion10/1
  Data Type Conversion10/1 -> IN_Port/1
  Compare To Constant9/1 -> Data Type Conversion11/1
  Data Type Conversion11/1 -> OUT_Port/1

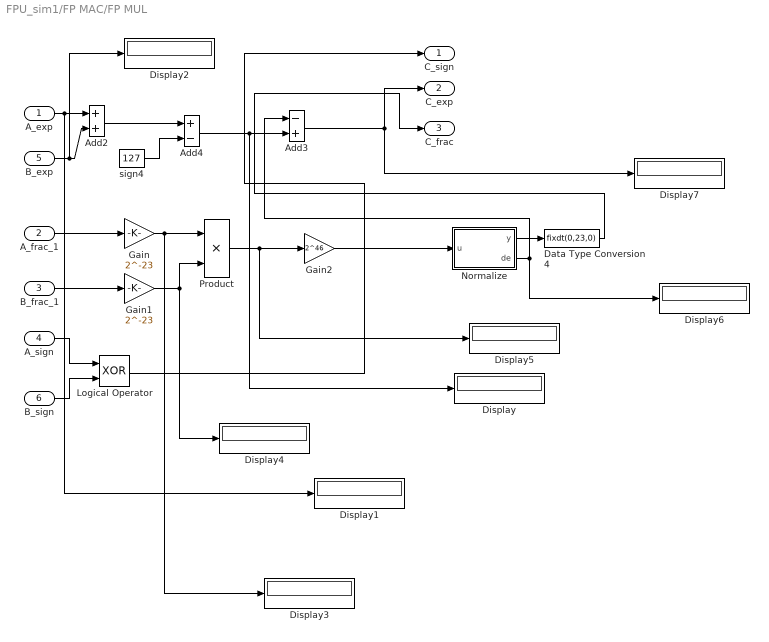
== system FPU_sim1/FP MAC/FP MUL ==
  A_exp : Inport  OutDataTypeStr=uint8
  A_frac_1 : Inport  Port=2  OutDataTypeStr=fixdt(0,24,0)
  B_frac_1 : Inport  Port=3  OutDataTypeStr=fixdt(0,24,0)
  A_sign : Inport  Port=4  OutDataTypeStr=boolean
  B_exp : Inport  Port=5  OutDataTypeStr=uint8
  B_sign : Inport  Port=6  OutDataTypeStr=boolean
  Add2 : Sum  OutDataTypeStr=fixdt(0,9,0)  RndMeth=Nearest
  Add3 : Sum  Inputs=-+  OutDataTypeStr=uint8  RndMeth=Nearest  SaturateOnIntegerOverflow=on
  Add4 : Sum  Inputs=+-  OutDataTypeStr=uint8  RndMeth=Nearest  SaturateOnIntegerOverflow=on
  Data Type Conversion4 : DataTypeConversion  OutDataTypeStr=fixdt(0,23,0)
  Display{,1..7} (8 alike) : Display
  Gain : Gain  Gain=2^-23  OutDataTypeStr=fixdt(0,24,23)  RndMeth=Nearest
  Gain1 : Gain  Gain=2^-23  OutDataTypeStr=fixdt(0,24,23)  RndMeth=Nearest
  Gain2 : Gain  Gain=2^46  OutDataTypeStr=fixdt(0,48,0)  RndMeth=Nearest
  Logical Operator : Logic  Operator=XOR  AllPortsSameDT=off  OutDataTypeStr=boolean
  Normalize : Stateflow chart  TreatAsAtomicUnit=on
  Product : Product  OutDataTypeStr=fixdt(0,48,46)  RndMeth=Nearest
  sign4 : Constant  Value=127  OutDataTypeStr=fixdt(0,9,0)
  C_sign : Outport  OutDataTypeStr=boolean
  C_exp : Outport  Port=2  OutDataTypeStr=uint8
  C_frac : Outport  Port=3  OutDataTypeStr=fixdt(0,23,0)
  wires:
  B_exp/1 -> Add2/2, Display2/1
  Normalize/1(y) -> Data Type Conversion4/1
  Normalize/2(de) -> Add3/1, Display6/1
  Add3/1 -> C_exp/1, Display7/1
  Data Type Conversion4/1 -> C_frac/1
  Logical Operator/1 -> C_sign/1
  Product/1 -> Display5/1, Gain2/1
  Add2/1 -> Add4/1
  sign4/1 -> Add4/2
  Add4/1 -> Add3/2, Display/1
  Gain/1 -> Product/1, Display3/1
  Gain1/1 -> Product/2, Display4/1
  A_frac_1/1 -> Gain/1
  B_frac_1/1 -> Gain1/1
  A_sign/1 -> Logical Operator/1
  A_exp/1 -> Add2/1, Display1/1
  B_sign/1 -> Logical Operator/2
  Gain2/1 -> Normalize/1(u)

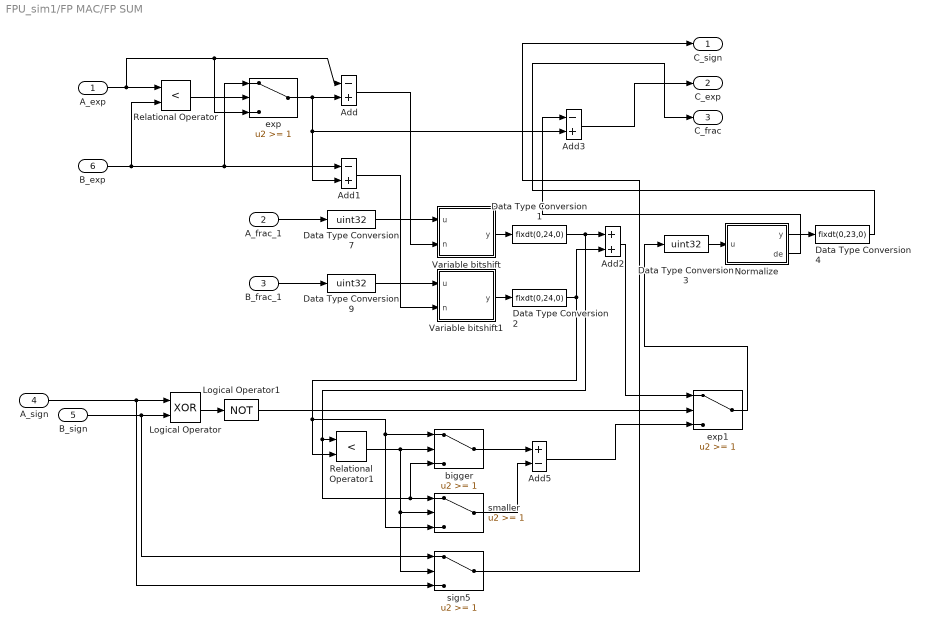
== system FPU_sim1/FP MAC/FP SUM ==
  A_exp : Inport  OutDataTypeStr=uint8
  A_frac_1 : Inport  Port=2  OutDataTypeStr=fixdt(0,24,0)
  B_frac_1 : Inport  Port=3  OutDataTypeStr=fixdt(0,24,0)
  A_sign : Inport  Port=4  OutDataTypeStr=boolean
  B_sign : Inport  Port=5  OutDataTypeStr=boolean
  B_exp : Inport  Port=6  OutDataTypeStr=uint8
  Add : Sum  Inputs=-+  OutDataTypeStr=int8
  Add1 : Sum  Inputs=-+  OutDataTypeStr=int8
  Add2 : Sum  OutDataTypeStr=fixdt(0,25,0)  RndMeth=Nearest
  Add3 : Sum  Inputs=-+  OutDataTypeStr=uint8  SaturateOnIntegerOverflow=on
  Add5 : Sum  Inputs=+-  OutDataTypeStr=fixdt(0,25,0)  RndMeth=Nearest
  Data Type Conversion1 : DataTypeConversion  OutDataTypeStr=fixdt(0,24,0)
  Data Type Conversion2 : DataTypeConversion  OutDataTypeStr=fixdt(0,24,0)
  Data Type Conversion3 : DataTypeConversion  OutDataTypeStr=uint32
  Data Type Conversion4 : DataTypeConversion  OutDataTypeStr=fixdt(0,23,0)
  Data Type Conversion7 : DataTypeConversion  OutDataTypeStr=uint32
  Data Type Conversion9 : DataTypeConversion  OutDataTypeStr=uint32
  Logical Operator : Logic  Operator=XOR  AllPortsSameDT=off  OutDataTypeStr=boolean
  Logical Operator1 : Logic  Operator=NOT  AllPortsSameDT=off  OutDataTypeStr=boolean
  Normalize : Stateflow chart  TreatAsAtomicUnit=on
  Relational Operator : RelationalOperator  Operator=<  OutDataTypeStr=boolean
  Relational Operator1 : RelationalOperator  Operator=<  OutDataTypeStr=boolean
  Variable bitshift : Stateflow chart  TreatAsAtomicUnit=on
  Variable bitshift1 : Stateflow chart  TreatAsAtomicUnit=on
  bigger : Switch  Threshold=1
  exp : Switch  Threshold=1
  exp1 : Switch  Threshold=1
  sign5 : Switch  Threshold=1
  smaller : Switch  Threshold=1
  C_sign : Outport  OutDataTypeStr=boolean
  C_exp : Outport  Port=2  OutDataTypeStr=uint8
  C_frac : Outport  Port=3  OutDataTypeStr=fixdt(0,23,0)
  wires:
  A_exp/1 -> Relational Operator/1, exp/3, Add/1
  B_exp/1 -> exp/1, Add1/1, Relational Operator/2
  A_frac_1/1 -> Data Type Conversion7/1
  Variable bitshift/1(y) -> Data Type Conversion1/1
  Data Type Conversion1/1 -> Add2/1, Relational Operator1/1, smaller/1, bigger/3
  Relational Operator/1 -> exp/2
  exp/1 -> Add/2, Add1/2, Add3/2
  B_frac_1/1 -> Data Type Conversion9/1
  Add/1 -> Variable bitshift/2(n)
  Add1/1 -> Variable bitshift1/2(n)
  Variable bitshift1/1(y) -> Data Type Conversion2/1
  Data Type Conversion2/1 -> Add2/2, Relational Operator1/2, bigger/1, smaller/3
  Add2/1 -> exp1/1
  Normalize/1(y) -> Data Type Conversion4/1
  Normalize/2(de) -> Add3/1
  Data Type Conversion3/1 -> Normalize/1(u)
  Data Type Conversion4/1 -> C_frac/1
  Logical Operator/1 -> Logical Operator1/1
  Logical Operator1/1 -> exp1/2
  Relational Operator1/1 -> bigger/2, smaller/2, sign5/2
  bigger/1 -> Add5/1
  smaller/1 -> Add5/2
  Add5/1 -> exp1/3
  exp1/1 -> Data Type Conversion3/1
  sign5/1 -> C_sign/1
  Data Type Conversion7/1 -> Variable bitshift/1(u)
  Data Type Conversion9/1 -> Variable bitshift1/1(u)
  A_sign/1 -> Logical Operator/1, sign5/3
  B_sign/1 -> Logical Operator/2, sign5/1
  Add3/1 -> C_exp/1

== system FPU_sim1/Embedded DSP in FPGA/IN_OUT_Controller/In_Port_Control ==
  In1 : Inport
  Enable : EnablePort
  Compare To Constant5 : simulink/Logic and Bit Operations/Compare To Constant  SystemSampleTime=-1  relop===  const=10  LogicOutDataTypeMode=boolean
  Compare To Constant6 : simulink/Logic and Bit Operations/Compare To Constant  SystemSampleTime=-1  relop===  const=11  LogicOutDataTypeMode=boolean
  FixPt Constant4 : Constant  DisableCoverage=on  OutDataTypeStr=fixdt(0,2,0)
  FixPt Constant5 : Constant  DisableCoverage=on  Value=2  OutDataTypeStr=fixdt(0,2,0)
  FixPt Constant6 : Constant  DisableCoverage=on  Value=0  OutDataTypeStr=fixdt(0,2,0)
  Switch5 : Switch  Criteria=u2 ~= 0
  Switch6 : Switch  Criteria=u2 ~= 0
  Out1 : Outport  InitialOutput=0
  wires:
  Switch6/1 -> Switch5/3
  FixPt Constant6/1 -> Switch6/3
  FixPt Constant5/1 -> Switch6/1
  FixPt Constant4/1 -> Switch5/1
  Compare To Constant6/1 -> Switch6/2
  Compare To Constant5/1 -> Switch5/2
  In1/1 -> Compare To Constant6/1, Compare To Constant5/1
  Switch5/1 -> Out1/1

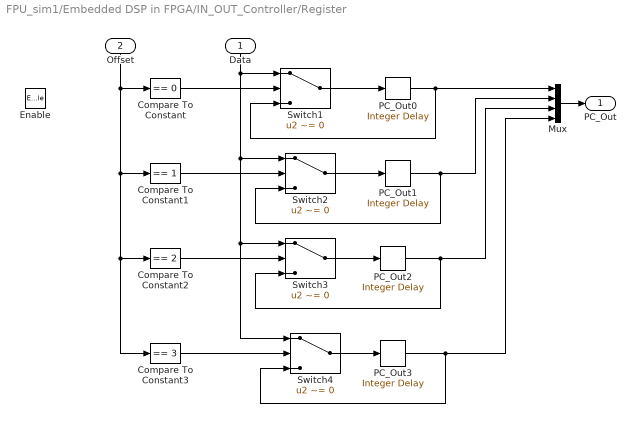
== system FPU_sim1/Embedded DSP in FPGA/IN_OUT_Controller/Register ==
  Data : Inport
  Offset : Inport  Port=2
  Enable : EnablePort
  Compare To Constant : simulink/Logic and Bit Operations/Compare To Constant  SystemSampleTime=-1  relop===  const=0  LogicOutDataTypeMode=boolean
  Compare To Constant1 : simulink/Logic and Bit Operations/Compare To Constant  SystemSampleTime=-1  relop===  const=1  LogicOutDataTypeMode=boolean
  Compare To Constant2 : simulink/Logic and Bit Operations/Compare To Constant  SystemSampleTime=-1  relop===  const=2  LogicOutDataTypeMode=boolean
  Compare To Constant3 : simulink/Logic and Bit Operations/Compare To Constant  SystemSampleTime=-1  relop===  const=3  LogicOutDataTypeMode=boolean
  Mux : Mux
  PC_Out{0..3} (4 alike) : simulink/Discrete/Integer Delay  NumDelays=1  vinit=0.0  samptime=-1
  Switch{1..4} (4 alike) : Switch  Criteria=u2 ~= 0
  PC_Out : Outport  InitialOutput=0
  wires:
  Mux/1 -> PC_Out/1
  Offset/1 -> Compare To Constant1/1, Compare To Constant3/1, Compare To Constant2/1, Compare To Constant/1
  Data/1 -> Switch4/1, Switch3/1, Switch2/1, Switch1/1
  Compare To Constant3/1 -> Switch4/2
  PC_Out3/1 -> Mux/4, Switch4/3
  Switch4/1 -> PC_Out3/1
  Compare To Constant2/1 -> Switch3/2
  PC_Out2/1 -> Mux/3, Switch3/3
  Switch3/1 -> PC_Out2/1
  Compare To Constant1/1 -> Switch2/2
  PC_Out1/1 -> Mux/2, Switch2/3
  Switch2/1 -> PC_Out1/1
  Compare To Constant/1 -> Switch1/2
  PC_Out0/1 -> Mux/1, Switch1/3
  Switch1/1 -> PC_Out0/1

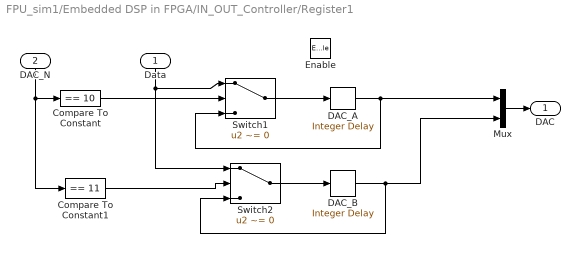
== system FPU_sim1/Embedded DSP in FPGA/IN_OUT_Controller/Register1 ==
  Data : Inport
  DAC_N : Inport  Port=2
  Enable : EnablePort
  Compare To Constant : simulink/Logic and Bit Operations/Compare To Constant  SystemSampleTime=-1  relop===  const=10  LogicOutDataTypeMode=boolean
  Compare To Constant1 : simulink/Logic and Bit Operations/Compare To Constant  SystemSampleTime=-1  relop===  const=11  LogicOutDataTypeMode=boolean
  DAC_A : simulink/Discrete/Integer Delay  NumDelays=1  vinit=0.0  samptime=-1
  DAC_B : simulink/Discrete/Integer Delay  NumDelays=1  vinit=0.0  samptime=-1
  Mux : Mux  Inputs=2
  Switch1 : Switch  Criteria=u2 ~= 0
  Switch2 : Switch  Criteria=u2 ~= 0
  DAC : Outport  InitialOutput=0
  wires:
  Switch1/1 -> DAC_A/1
  DAC_A/1 -> Switch1/3, Mux/1
  Compare To Constant/1 -> Switch1/2
  Switch2/1 -> DAC_B/1
  DAC_B/1 -> Switch2/3, Mux/2
  Compare To Constant1/1 -> Switch2/2
  Data/1 -> Switch1/1, Switch2/1
  DAC_N/1 -> Compare To Constant/1, Compare To Constant1/1
  Mux/1 -> DAC/1

== system FPU_sim1/Embedded DSP in FPGA/IN_OUT_Controller/Rise_detect ==
  In1 : Inport
  BRAM3 : simulink/Discrete/Integer Delay  NumDelays=1  vinit=0.0  samptime=-1
  Logical Operator1 : Logic  AllPortsSameDT=off  OutDataTypeStr=boolean
  Logical Operator6 : Logic  Operator=NOT  AllPortsSameDT=off  OutDataTypeStr=boolean
  Out1 : Outport
  wires:
  Logical Operator1/1 -> Out1/1
  In1/1 -> Logical Operator1/2, BRAM3/1
  BRAM3/1 -> Logical Operator6/1
  Logical Operator6/1 -> Logical Operator1/1

== system FPU_sim1/Embedded DSP in FPGA/IN_OUT_Controller/Rise_detect1 ==
  In1 : Inport
  BRAM3 : simulink/Discrete/Integer Delay  NumDelays=1  vinit=0.0  samptime=-1
  Logical Operator1 : Logic  AllPortsSameDT=off  OutDataTypeStr=boolean
  Logical Operator6 : Logic  Operator=NOT  AllPortsSameDT=off  OutDataTypeStr=boolean
  Out1 : Outport
  wires:
  Logical Operator6/1 -> Logical Operator1/1
  BRAM3/1 -> Logical Operator6/1
  In1/1 -> BRAM3/1, Logical Operator1/2
  Logical Operator1/1 -> Out1/1

== matlab function 4 to 1 ==
  data: out_d output uint32; in_d input uint8 size=4
function out_d  = fcn(in_d)
%#eml
out_d=uint32(bitor(bitor(bitor(in_d(1),bitshift(in_d(2),8)),bitshift(in_d(3),16)),bitshift(in_d(4),24)));

== matlab function Block RAM/Embedded MATLAB Function ==
  data: adr input double; d_out output uint32; we input double; d_in input double; mem input double size=2048; mem_o output double size=2048
function [d_out,mem_o] = fcn(adr,we,d_in,mem)
%#eml

if (adr<2048)
        d_out=uint32(mem(adr+1));
    if (we==1)
        mem(adr+1)=d_in;
    end
else
    d_out=uint32(0);
end
mem_o=mem;

== matlab function FP MAC/FP SUM/Normalize ==
  data: u input uint32; y output uint32; de output double
function [y,de] = fcn(u)
%#eml

buf=u;
p=int8(-1);
c=bitand(buf,2^24);
for ind=1:25
    if (~c)
        p=p+1;
        buf=bitshift(buf,1);
        c=bitand(buf,2^24);
    end
end
bufy = bitand(bitshift(u,p),2^23-1);
y=bufy;
de=p;

== matlab function FP MAC/FP SUM/Variable bitshift ==
  data: u input uint32; y output uint32; n input int8
function y = fcn(u,n)
%#eml

y = bitshift(u,-n);

== matlab function 1 to 4 ==
  data: out_d output uint8; in_d input uint32
function out_d  = fcn(in_d)
%#eml
out_d=typecast(in_d,'uint8');

== matlab function FP MAC/FP SUM/Variable bitshift1 ==
  data: u input uint32; y output uint32; n input int8
function y = fcn(u,n)
%#eml

y = bitshift(u,-n);

== matlab function Block RAM/1 to 1 ==
  data: out_d output single; in_d input uint32 size=1
function out_d  = fcn(in_d)
%#eml
out_d=typecast(in_d,'single');

== matlab function FP MAC/FP MUL/Normalize ==
  data: u input fixdt(0,48,0); y output uint32; de output double
function [y,de] = fcn(u)
%#eml

buf=u;
p=int8(-1);
c=bitand(buf,fi(2^47,0,48,0));
for ind=1:25
    if (c==0)
        p=p+1;
        buf=bitshift(buf,1);
        c=bitand(buf,fi(2^47,0,48,0));
    end
end
bufy = bitand(bitshift(u,p),fi(2^46-1,0,48,0));
y=uint32(bitshift(bufy,-23));
de=p;

== matlab function Block RAM/1 to 2 ==
  data: out_d output single; in_d input uint32 size=1
function out_d  = fcn(in_d)
%#eml
out_d=typecast(in_d,'single');

== matlab function FP MAC/FP Extract ==
  data: u input uint32; sig output uint8; exp output uint8; frac output uint32
function [sig,exp,frac] = fcn(u)
%#eml

z=u;
sig=uint8(bitshift(z,-31));
exp=uint8(bitshift(bitshift(z,1),-24));
frac=uint32(bitand(z,8388607));
%bexp=uint8(bitshift(bitshift(z,1),-23));
% exp1=uint8(zeros(8,1));
% frac1=uint8(zeros(23,1));
% for ind=0:7
%     exp1(ind+1)=uint8(bitand(bitshift(bexp,-ind),1));
% end
% bfrac=z;
% for ind=0:22
%     frac1(ind+1)=uint8(bitand(bitshift(bfrac,-ind),1));
% end
% exp=exp1;
% frac=frac1;

== matlab function FP MAC/FP Extract1 ==
  data: u input uint32; sig output uint8; exp output uint8; frac output uint32
function [sig,exp,frac] = fcn(u)
%#eml

z=u;
sig=uint8(bitshift(z,-31));
exp=uint8(bitshift(bitshift(z,1),-24));
frac=uint32(bitand(z,8388607));
%bexp=uint8(bitshift(bitshift(z,1),-23));
% exp1=uint8(zeros(8,1));
% frac1=uint8(zeros(23,1));
% for ind=0:7
%     exp1(ind+1)=uint8(bitand(bitshift(bexp,-ind),1));
% end
% bfrac=z;
% for ind=0:22
%     frac1(ind+1)=uint8(bitand(bitshift(bfrac,-ind),1));
% end
% exp=exp1;
% frac=frac1;

== matlab function FP MAC/FP Extract2 ==
  data: u input uint32; sig output uint8; exp output uint8; frac output uint32
function [sig,exp,frac] = fcn(u)
%#eml

z=u;
sig=uint8(bitshift(z,-31));
exp=uint8(bitshift(bitshift(z,1),-24));
frac=uint32(bitand(z,8388607));
%bexp=uint8(bitshift(bitshift(z,1),-23));
% exp1=uint8(zeros(8,1));
% frac1=uint8(zeros(23,1));
% for ind=0:7
%     exp1(ind+1)=uint8(bitand(bitshift(bexp,-ind),1));
% end
% bfrac=z;
% for ind=0:22
%     frac1(ind+1)=uint8(bitand(bitshift(bfrac,-ind),1));
% end
% exp=exp1;
% frac=frac1;

== matlab function FP MAC/FP Compose ==
  data: sig input uint8; exp input uint8; frac input uint32; y output uint32
function y = fcn(sig,exp,frac)
%#eml

z=uint32(0);
if sig
    z=uint32(bitshift(uint32(1),31));
end
buf=uint32(bitshift(uint32(exp),23));
z=bitor(z,buf);
z=bitor(z,frac);
y=z;

== matlab function 4 to 2 ==
  data: y output single; u input uint32
function y  = fcn(u)
%#eml
y=typecast(u,'single');

== matlab function 4 to 3 ==
  data: y output uint32; u input single
function y  = fcn(u)
%#eml
y=typecast(u,'uint32');

== matlab function 4 to 4 ==
  data: y output uint32; u input single
function y  = fcn(u)
%#eml
y=typecast(u,'uint32');

== matlab function 4 to 5 ==
  data: y output uint32; u input single
function y  = fcn(u)
%#eml
y=typecast(u,'uint32');

== matlab function FP MAC/4 to 2 ==
  data: y output single; u input uint32
function y  = fcn(u)
%#eml
y=typecast(u,'single');

== matlab function FP MAC/FP Compose1 ==
  data: sig input uint8; exp input uint8; frac input uint32; y output uint32
function y = fcn(sig,exp,frac)
%#eml

z=uint32(0);
if sig
    z=uint32(bitshift(uint32(1),31));
end
buf=uint32(bitshift(uint32(exp),23));
z=bitor(z,buf);
z=bitor(z,frac);
y=z;

== matlab function 4 to 6 ==
  data: y output single; u input uint32
function y  = fcn(u)
%#eml
y=typecast(u,'single');

== matlab function 4 to 7 ==
  data: y output single; u input uint32
function y  = fcn(u)
%#eml
y=typecast(u,'single');

== matlab function Embedded DSP in FPGA/4 to 7 ==
  data: y output single; u input uint32
function y  = fcn(u)
%#eml
y=typecast(u,'single');

== matlab function 4 to 8 ==
  data: y output single; u input uint32
function y  = fcn(u)
%#eml
y=typecast(u,'single');

== matlab function 4 to 9 ==
  data: y output uint32; u input single
function y  = fcn(u)
%#eml
y=typecast(u,'uint32');
